simulink model "ChuaMultipleSynch_MPC"  (R2014b)
settings: Solver=ode4  StartTime=0.0  StopTime=T  FixedStep=Ts  RelTol=1e-8
values from neighbouring files (symbols this model uses):
  mpc = MPCController(model, N)    [main_mpc.m]
  Ts = T/N    (= 0.01)    [PlotEig.m]    (also in main_mpc.m; main_sim.m)
  x0 = [0.02;0.05;0.04;0.0;1.0;0.0]    [PlotEig.m]    (also in main_mpc.m; main_sim.m)
undefined symbols (not defined in the file or in its folder): MPC_Controller
settings Model: Creator=gianni  LastModifiedBy=Gianni

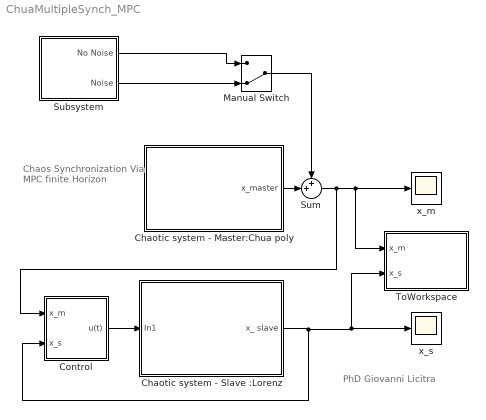
== system ChuaMultipleSynch_MPC ==
  note: PhD Giovanni Licitra
  note: Chaos Synchronization
      | Via MPC finite Horizon
  Chaotic system - Master:Chua poly : Subsystem
      mask Display: image('Chaos.jpg')
  Chaotic system - Slave :Lorenz : Subsystem
      mask Display: image('Chaos.jpg')
  Control : Subsystem
  Manual Switch : ManualSwitch  CurrentSetting=0
  Subsystem : Subsystem
  Sum : Sum  Inputs=++|
  ToWorkspace : Subsystem
  x_m : Scope
      settings: YMin=-0.4  YMax=0.4
  x_s : Scope
      settings: YMin=-2
  wires:
  Control/1(u(t)) -> Chaotic system - Slave :Lorenz/1(In1)
  Sum/1 -> ToWorkspace/1(x_m), x_m/1, Control/1(x_m)
  Chaotic system - Slave :Lorenz/1(x_ slave) -> Control/2(x_s), ToWorkspace/2(x_s), x_s/1
  Chaotic system - Master:Chua poly/1(x_master) -> Sum/2
  Manual Switch/1 -> Sum/1
  Subsystem/1(No Noise) -> Manual Switch/1
  Subsystem/2(Noise) -> Manual Switch/2

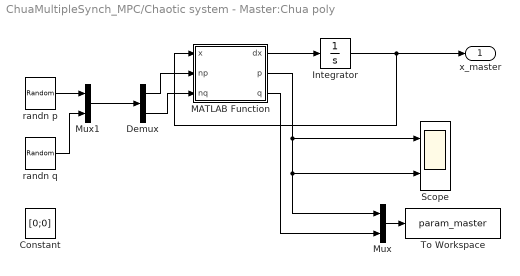
== system ChuaMultipleSynch_MPC/Chaotic system - Master:Chua poly ==
  Constant : Constant  Value=[0;0]
  Demux : Demux  Outputs=2
  Integrator : Integrator  InitialCondition=x0([1:3])
  MATLAB Function : MATLAB Function  TreatAsAtomicUnit=on
  Mux : Mux  Inputs=2
  Mux1 : Mux  Inputs=2
  Scope : Scope  NumInputPorts=2
      settings: YMin=9.5~13.6  YMax=10.5~14.8  SaveName=ScopeData5
  To Workspace : ToWorkspace  VariableName=param_master  SaveFormat=Timeseries  SampleTime=-1
  randn p : UniformRandomNumber  Minimum=-0.5  Maximum=0.5  SampleTime=Ts
  randn q : UniformRandomNumber  Minimum=-0.5  Maximum=0.5  SampleTime=Ts
  x_master : Outport
  wires:
  Integrator/1 -> MATLAB Function/1(x), x_master/1
  MATLAB Function/1(dx) -> Integrator/1
  Mux/1 -> To Workspace/1
  randn p/1 -> Mux1/1
  randn q/1 -> Mux1/2
  Demux/1 -> MATLAB Function/2(np)
  Demux/2 -> MATLAB Function/3(nq)
  Mux1/1 -> Demux/1
  MATLAB Function/2(p) -> Scope/1, Scope/2, Mux/1
  MATLAB Function/3(q) -> Mux/2

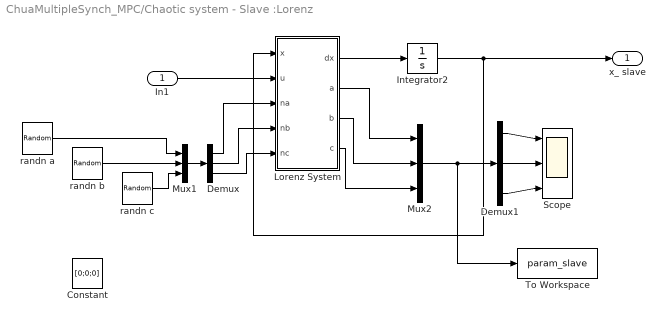
== system ChuaMultipleSynch_MPC/Chaotic system - Slave :Lorenz ==
  In1 : Inport
  Constant : Constant  Value=[0;0;0]
  Demux : Demux  Outputs=3
  Demux1 : Demux  Outputs=3
  Integrator2 : Integrator  InitialCondition=x0([4:6])
  Lorenz System : MATLAB Function  TreatAsAtomicUnit=on
  Mux1 : Mux  Inputs=3
  Mux2 : Mux  Inputs=3
  Scope : Scope  NumInputPorts=3
      settings: YMin=9.5~13.6~-5  YMax=10.5~14.8~5  SaveName=ScopeData6
  To Workspace : ToWorkspace  VariableName=param_slave  SaveFormat=Timeseries  SampleTime=-1
  randn a : UniformRandomNumber  Minimum=-0.5  Maximum=0.5  SampleTime=Ts
  randn b : UniformRandomNumber  Minimum=-0.5  Maximum=0.5  SampleTime=Ts
  randn c : UniformRandomNumber  Minimum=-0.5  Maximum=0.5  SampleTime=Ts
  x_ slave : Outport
  wires:
  Lorenz System/1(dx) -> Integrator2/1
  In1/1 -> Lorenz System/2(u)
  Integrator2/1 -> x_ slave/1, Lorenz System/1(x)
  randn a/1 -> Mux1/1
  randn b/1 -> Mux1/2
  Demux/1 -> Lorenz System/3(na)
  Demux/2 -> Lorenz System/4(nb)
  Mux1/1 -> Demux/1
  randn c/1 -> Mux1/3
  Demux/3 -> Lorenz System/5(nc)
  Lorenz System/2(a) -> Mux2/1
  Lorenz System/3(b) -> Mux2/2
  Lorenz System/4(c) -> Mux2/3
  Demux1/1 -> Scope/1
  Demux1/2 -> Scope/2
  Demux1/3 -> Scope/3
  Mux2/1 -> To Workspace/1, Demux1/1

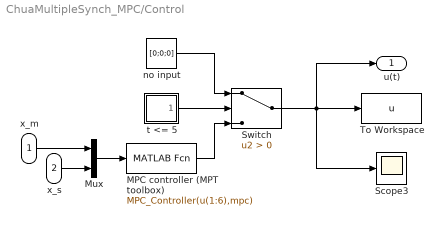
== system ChuaMultipleSynch_MPC/Control ==
  x_m : Inport
  x_s : Inport  Port=2
  MPC controller (MPT toolbox) : MATLABFcn  MATLABFcn=MPC_Controller(u(1:6),mpc)
  Mux : Mux  Inputs=2
  Scope3 : Scope
      settings: YMin=-10  YMax=10  SaveName=ScopeData3
  Switch : Switch  Criteria=u2 > Threshold
  To Workspace : ToWorkspace  VariableName=u  SaveFormat=Timeseries  SampleTime=-1
  no input : Constant  Value=[0;0;0]
  t <= 5 : Subsystem
  u(t) : Outport
  wires:
  x_s/1 -> Mux/2
  x_m/1 -> Mux/1
  t <= 5/1(t <= 3) -> Switch/2
  no input/1 -> Switch/1
  Switch/1 -> Scope3/1, To Workspace/1, u(t)/1
  MPC controller (MPT toolbox)/1 -> Switch/3
  Mux/1 -> MPC controller (MPT toolbox)/1

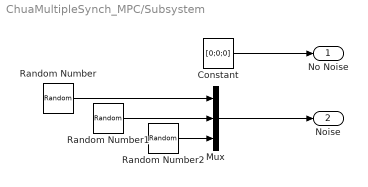
== system ChuaMultipleSynch_MPC/Subsystem ==
  Constant : Constant  Value=[0;0;0]
  Mux : Mux  Inputs=3
  Random Number : RandomNumber  Variance=0.001
  Random Number1 : RandomNumber  Variance=0.001
  Random Number2 : RandomNumber  Variance=0.001
  No Noise : Outport
  Noise : Outport  Port=2
  wires:
  Mux/1 -> Noise/1
  Random Number/1 -> Mux/1
  Random Number1/1 -> Mux/2
  Random Number2/1 -> Mux/3
  Constant/1 -> No Noise/1

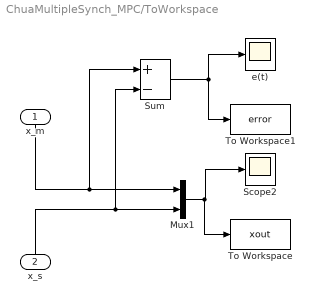
== system ChuaMultipleSynch_MPC/ToWorkspace ==
  x_m : Inport
  x_s : Inport  Port=2
  Mux1 : Mux  Inputs=2
  Scope2 : Scope
      settings: YMin=-20  YMax=50  SaveName=ScopeData2
  Sum : Sum  Inputs=+-
  To Workspace : ToWorkspace  VariableName=xout  SaveFormat=Timeseries  SampleTime=-1
  To Workspace1 : ToWorkspace  VariableName=error  SaveFormat=Timeseries  SampleTime=-1
  e(t) : Scope
      settings: YMin=-50  YMax=20  SaveName=ScopeData4
  wires:
  Mux1/1 -> To Workspace/1, Scope2/1
  x_s/1 -> Sum/2, Mux1/2
  x_m/1 -> Sum/1, Mux1/1
  Sum/1 -> To Workspace1/1, e(t)/1

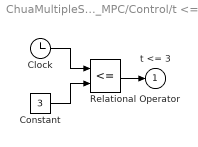
== system ChuaMultipleSynch_MPC/Control/t <= 5 ==
  Clock : Clock
  Constant : Constant  Value=3
  Relational Operator : RelationalOperator  Operator=<=  InputSameDT=on
  t <= 3 : Outport  InitialOutput=0
  wires:
  Constant/1 -> Relational Operator/2
  Clock/1 -> Relational Operator/1
  Relational Operator/1 -> t <= 3/1

== matlab function ChuaMultipleSynch_MPC/Chaotic system - Master:Chua poly/MATLAB Function ==
  data: x input; dx output; np input; nq input; p output; q output
function [dx,p,q] = ode(x,np,nq)                           
    % master: chua's circuit poly    
    p = 10+np;
    q = 100/7+nq;                  % slave system parameter    
    x1 = x(1);y1 = x(2);z1 = x(3);     % master sys states  
    f_x1 = 2*x1^3 - x1/7;              % non linearity master sys
   
    dx = [p*(y1-f_x1);   % Chua poly : f1        
          x1-y1+z1;      % Chua poly : f2
          -q*y1          % Chua poly : f3
          ];       
end

== matlab function ChuaMultipleSynch_MPC/Chaotic system - Slave :Lorenz/Lorenz System ==
  data: x input; dx output; u input; na input; nb input; nc input; a output; b output; c output
function [dx,a,b,c] = ode(x,u,na,nb,nc)                             
    % slave : Lorenz System
    a = 28+na;
    b = 10+nb;
    c = 8/3+nc;             % master system parameter
    x2 = x(1);y2 = x(2);z2 = x(3);     % slave sys states
    ux = u(1);uy = u(2); uz = u(3);    % control to slave system
   
    dx = [b*(y2-x2)+ ux;      % Lorenz : f1 
          x2*(a-z2)-y2 + uy;  % Lorenz : f2
          x2*y2-c*z2 + uz     % Lorenz : f3
          ];          
end
